simulink model "sl_onelink_control_compatible"  (R2015a)
settings: Solver=ode45  SolverMode=SingleTasking  StartTime=0.0  StopTime=10.0  RelTol=1e-3
libraries: roblocks x2
settings Model: CovMetricSettings=dwe  CovHtmlReporting=off  covSaveCumulativeToWorkspaceVar=off  CovSaveSingleToWorkspaceVar=off  CovExternalEMLEnable=on  Creator=mkillpack  LastModifiedBy=mkillpack
settings DataIOCC: LimitDataPoints=off  SaveFormat=Dataset
settings DebuggingCC: SFUnexpectedBacktrackingDiag=error  SFNoUnconditionalDefaultTransitionDiag=error
settings HardwareCC: ProdBitPerPointer=64  ProdLargestAtomicFloat=Float  ProdIntDivRoundTo=Zero  ProdEndianess=LittleEndian  ProdHWDeviceType=Specified
settings ModelReferenceCC: PropagateSignalLabelsOutOfModel=on
settings GRTTargetCC: TargetLangStandard=C99 (ISO)  GeneratePreprocessorConditionals=Use local settings

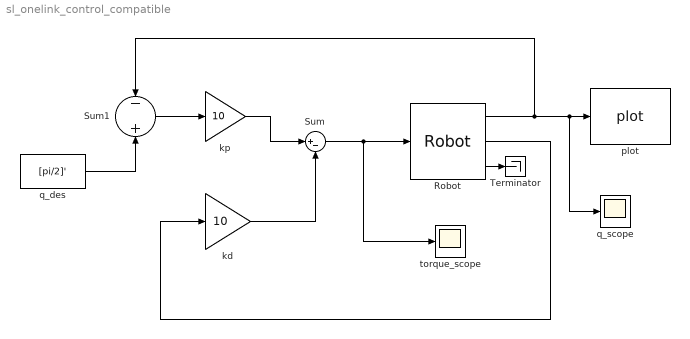
== system sl_onelink_control_compatible ==
  Robot : roblocks/Dynamics/Robot  robot=onelink  q0=[0]
  Sum : Sum  Inputs=|+-
  Sum1 : Sum  Inputs=-|+
  Terminator : Terminator
  kd : Gain  Gain=10
  kp : Gain  Gain=10
  plot : roblocks/Robot Graphics/plot  robot=onelink  fps=25  holdplot=on
  q_des : Constant  Value=[pi/2]'
  q_scope : Scope
      settings: TimeRange=auto  MaxDataPoints=5000  SaveToWorkspace=off  YMin=-0.19634  YMax=1.7671  SampleTime=-1
  torque_scope : Scope
      settings: TimeRange=auto  MaxDataPoints=5000  SaveToWorkspace=off  SaveName=ScopeData  YMin=-2.78936  YMax=17.76322  SampleTime=-1
  wires:
  Robot/1 -> Sum1/1, q_scope/1, plot/1
  Sum1/1 -> kp/1
  kp/1 -> Sum/1
  Robot/2 -> kd/1
  kd/1 -> Sum/2
  Sum/1 -> torque_scope/1, Robot/1
  q_des/1 -> Sum1/2
  Robot/3 -> Terminator/1
